simulink model "PubIfCommonEHRV2_MDL"  (R2020b)
settings: Solver=FixedStepAuto  StartTime=0.0  StopTime=Inf  RelTol=1e-3
PostLoadFcn:
  | if any(exist('dsrtsu_mdlpostloadfcn', 'file') ~= 0), dsrtsu_mdlpostloadfcn('Execute', bdroot); end
InitFcn:
  | , if any(exist('dsmpb_private', 'file') ~= 0), dsmpb_private('dsmpb_mdlclblib', 'Init', bdroot); end,
undefined symbols (not defined in the file): CAMERA_STATE_INITIAL, CAMERA_STATE_NORMAL, CURVATURE_UNKNOWN, DISTANCE_UNKONWN, DRIVING_ON_HIGHWAY_YES, EHR_CYCLE, FORWARD_LOOKING_DISTANCE_LIMIT, IFC_HUT_INTERFACE_NO_RESPONSE, IFC_HUT_INTERFACE_RESPONSE, MAP_DATA_VALID_VALID, MSG_TYPE_PROFILE_LONG, MSG_TYPE_PROFILE_SHORT, MSG_TYPE_SEGMENT, MSG_TYPE_STUB, OFFSET_INVALID, OFFSET_MAX, P_EHRV2_dCurvatureFar, P_EHRV2_dCurvatureMatrix, P_EHRV2_dSlopeFar, P_EHRV2_dSlopeMatrix, P_EHRV2_dVehForwardLooking, P_EHRV2_dVehRearLooking, P_EHRV2_tIFCHUTNoResponseOfForecastTreeReset, P_EHRV2_tIFCHUTNoResponseOfTimeout, P_EHRV2_tIFCHUTResponseTimeout, PROFILE_SHORT_NO_OTHER_VALUE, PROFILE_SHORT_TYPE_CURVATURE, PROFILE_SHORT_TYPE_SLOPE, REAR_LOOKING_DISTANCE_LIMIT, SLOPE_UNKNOWN, STUB_CMPLX_INSCT, STUB_FORM_OF_WAY_HIGH_RING_ROAD, STUB_FORM_OF_WAY_NORMAL_RING_ROAD
libraries: simulink x5
(part 2 of 4)

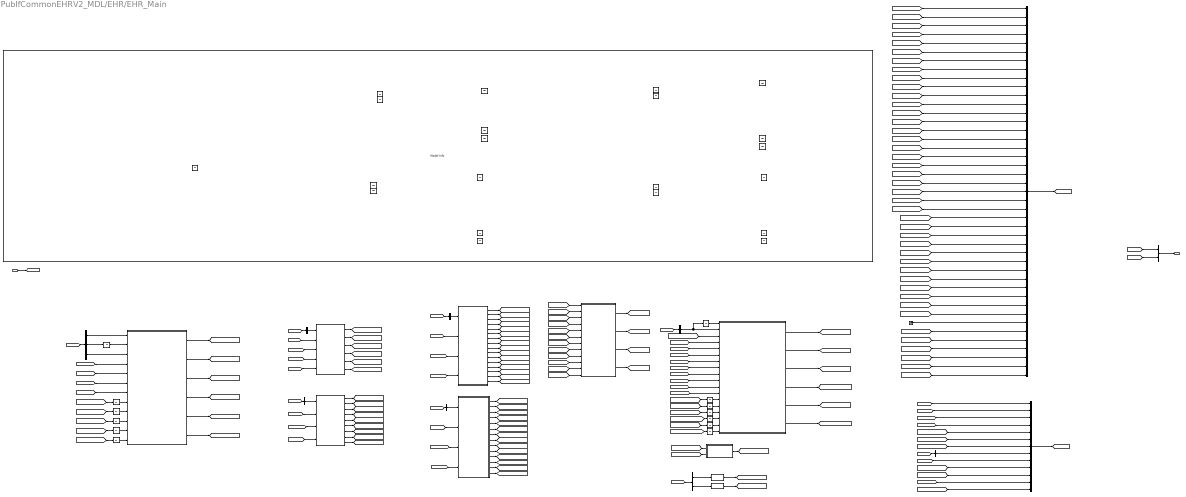
== system PubIfCommonEHRV2_MDL/EHR/EHR_Main ==
  EHR_InputData : Inport
  Bus Creator : BusCreator  Inputs=43
  Bus Creator1 : BusCreator  Inputs=13
  Bus Creator2 : BusCreator  Inputs=2
  Bus Selector : BusSelector  OutputSignals=PositionStruct,PositionStruct,StubStruct
  Bus Selector1 : BusSelector  OutputSignals=SegmentStruct
  Bus Selector10 : BusSelector  OutputSignals=PositionStruct,ProfileShortStruct
  Bus Selector11 : BusSelector  OutputSignals=PositionStruct,PositionStruct,ProfileShortStruct
  Bus Selector12 : BusSelector  OutputSignals=ProfileLongStruct
  Bus Selector13 : BusSelector  OutputSignals=PositionStruct,ProfileLongStruct
  Bus Selector14 : BusSelector  OutputSignals=PositionStruct,PositionStruct,ProfileLongStruct
  Bus Selector{6,8,15..16} (4 alike) : BusSelector  OutputSignals=PositionStruct
  Bus Selector17 : BusSelector  OutputSignals=OtherMessageStruct.ECU_State
  Bus Selector18 : BusSelector  OutputSignals=PositionStruct,PositionStruct,OtherMessageStruct.VehSpdDisp
  Bus Selector19 : BusSelector  OutputSignals=StubStruct
  Bus Selector2 : BusSelector  OutputSignals=StubStruct
  Bus Selector20 : BusSelector  OutputSignals=MetaDataStruct.MetaSpdUnits,MetaDataStruct.MetaCountryCode
  Bus Selector3 : BusSelector  OutputSignals=PositionStruct,StubStruct
  Bus Selector4 : BusSelector  OutputSignals=PositionStruct,SegmentStruct
  Bus Selector5 : BusSelector  OutputSignals=PositionStruct,PositionStruct,SegmentStruct
  Bus Selector7 : BusSelector  OutputSignals=SegmentStruct.SegMsgType
  Bus Selector9 : BusSelector  OutputSignals=ProfileShortStruct
  DR_Calc_IFCHUTInterface : MATLAB Function  TreatAsAtomicUnit=on
  DR_Calc_MapDataValid : MATLAB Function  TreatAsAtomicUnit=on
  DR_Calc_ProfileLongReconstruct : MATLAB Function  TreatAsAtomicUnit=on
  DR_Calc_ProfileShortReconstruct : MATLAB Function  TreatAsAtomicUnit=on
  DR_Calc_RampDistance : MATLAB Function  TreatAsAtomicUnit=on
  DR_Calc_SegmentReconstruct : MATLAB Function  TreatAsAtomicUnit=on
  DR_Calc_StubReconstruct : MATLAB Function  TreatAsAtomicUnit=on
  DS_Calc_ForecastTreeReset : MATLAB Function  TreatAsAtomicUnit=on
  DS_Calc_ProfileLongIsInDataWindow : MATLAB Function  TreatAsAtomicUnit=on
  DS_Calc_ProfileLongIsUpdated : MATLAB Function  TreatAsAtomicUnit=on
  DS_Calc_ProfileLongVector : MATLAB Function  TreatAsAtomicUnit=on
  DS_Calc_ProfileShortIsInDataWindow : MATLAB Function  TreatAsAtomicUnit=on
  DS_Calc_ProfileShortIsUpdated : MATLAB Function  TreatAsAtomicUnit=on
  DS_Calc_ProfileShortVector : MATLAB Function  TreatAsAtomicUnit=on
  DS_Calc_SegmentIsInDataWindow : MATLAB Function  TreatAsAtomicUnit=on
  DS_Calc_SegmentIsUpdated : MATLAB Function  TreatAsAtomicUnit=on
  DS_Calc_SegmentVector : MATLAB Function  TreatAsAtomicUnit=on
  DS_Calc_StubIsInDataWindow : MATLAB Function  TreatAsAtomicUnit=on
  DS_Calc_StubIsUpdated : MATLAB Function  TreatAsAtomicUnit=on
  DS_Calc_StubVector : MATLAB Function  TreatAsAtomicUnit=on
  Data Type Conversion : DataTypeConversion  OutDataTypeStr=uint8
  Data Type Conversion1 : DataTypeConversion  OutDataTypeStr=uint16
  Ground11 : Ground
  MATLAB Function : MATLAB Function  TreatAsAtomicUnit=on
  Model Info1 : simulink/Model-Wide Utilities/Model Info  Frame=on  DisplayStringWithTags=DS_Calc_SegmentVector  HorizontalTextAlignment=Left  LeftAlignmentValue=0.02
  Model Info2 : simulink/Model-Wide Utilities/Model Info  Frame=on  DisplayStringWithTags=DS_Calc_ProfileShortVector  HorizontalTextAlignment=Left  LeftAlignmentValue=0.02
  Model Info3 : simulink/Model-Wide Utilities/Model Info  Frame=on  DisplayStringWithTags=DS_Calc_StubVector  HorizontalTextAlignment=Left  LeftAlignmentValue=0.02
  Model Info4 : simulink/Model-Wide Utilities/Model Info  Frame=on  DisplayStringWithTags=DS_Calc_ProfileLongVector  HorizontalTextAlignment=Left  LeftAlignmentValue=0.02
  Model Info9 : simulink/Model-Wide Utilities/Model Info  Frame=on  DisplayStringWithTags=DS  HorizontalTextAlignment=Left  LeftAlignmentValue=0.02
  Unit Delay{,1..33} (34 alike) : UnitDelay  SampleTime=-1  HasFrameUpgradeWarning=on
  EHR_OutputData : Outport
  wires:
  DR_Calc_ProfileLongReconstruct/1(RampInDistance) -> [RampInDistance2]
  [IFCHUTInterfaceNoResponseFlag1] -> Unit Delay20/1
  Unit Delay6/1 -> DS_Calc_ProfileShortIsUpdated/2(ProfileShortVector)
  Bus Selector3/2 -> DS_Calc_StubIsInDataWindow/2(StubStruct)  "<StubStruct>"
  Unit Delay30/1 -> DS_Calc_ForecastTreeReset/2(StubStructK1)
  DS_Calc_StubVector/2(StubVectorSize) -> [StubVectorSize]  "EHRV2_StubVectorSize"
  [StubVectorSize] -> DR_Calc_StubReconstruct/3(StubVectorSize)
  Bus Selector18/2 -> Unit Delay31/1  "<PositionStruct>"
  Bus Selector19/1 -> Unit Delay30/1, DS_Calc_ForecastTreeReset/1(StubStruct)  "<StubStruct>"
  [PositionPathIdxInvalidCycles] -> Unit Delay29/1
  [SegmentVectorSize] -> Unit Delay15/1
  [MapDataValid] -> DR_Calc_ProfileLongReconstruct/4(MapDataValid)
  [MapDataValid] -> DR_Calc_ProfileShortReconstruct/4(MapDataValid)
  [SegmentVectorSize] -> DR_Calc_MapDataValid/5(SegmentVectorSize)
  DR_Calc_MapDataValid/3(PositionJumpOutOfRange) -> [PositionJumpOutOfRange]  "EHRV2_PositionJumpOutOfRange"
  Bus Selector3/1 -> DS_Calc_StubIsInDataWindow/1(PositionStruct)  "<PositionStruct>"
  [EHR_InputData] -> Bus Selector4/1
  [StubVectorSize] -> DS_Calc_ProfileShortVector/8(StubVectorSize)
  DS_Calc_ForecastTreeReset/1(ForecastTreeResetFlag) -> [ForecastTreeResetFlag]  "EHRV2_ForecastTreeResetFlag"
  Unit Delay8/1 -> DS_Calc_StubIsUpdated/3(StubVectorSize)
  [ProfileShortVectorSize] -> DR_Calc_MapDataValid/6(ProfileShortVectorSize)
  Bus Selector5/2 -> Unit Delay3/1  "<PositionStruct>"
  Bus Selector18/3 -> DR_Calc_MapDataValid/3(IPVehSpdDisp)  "<VehSpdDisp>"
  DR_Calc_MapDataValid/4(PositionJumpOutOfRangeCycles) -> [PositionJumpOutOfRangeCycles]  "EHRV2_PositionJumpOutOfRangeCycles"
  [ProfileLongIsUpdated] -> DS_Calc_ProfileLongVector/4(ProfileLongIsUpdated)
  [MapDataValid] -> DR_Calc_StubReconstruct/4(MapDataValid)
  [ForecastTreeResetFlag] -> Bus Creator1/12  "ForecastTreeResetFlag"
  DR_Calc_ProfileShortReconstruct/5(RoadSlopeFar) -> [RoadSlopeFar]
  [StubVectorSize] -> Unit Delay8/1
  [StubVectorSize] -> Unit Delay2/1
  Bus Selector13/1 -> DS_Calc_ProfileLongIsInDataWindow/1(PositionStruct)  "<PositionStruct>"
  [RoadSlopeMatrix] -> Bus Creator/35  "RoadSlopeMatrix"
  Unit Delay14/1 -> DS_Calc_SegmentIsUpdated/2(SegmentVector)
  [ForecastTreeResetFlag] -> DS_Calc_StubVector/6(ForecastTreeResetFlag)
  [StubVector] -> DR_Calc_StubReconstruct/2(StubVector)
  DR_Calc_ProfileShortReconstruct/6(RoadCurvatureMatrix) -> [RoadCurvatureMatrix]
  [NumOfLaneDrvDir] -> Bus Creator/10  "NumOfLaneDrvDir"
  DR_Calc_MapDataValid/2(PositionOffsetCycles) -> [PositionOffsetCycles]  "EHRV2_PositionOffsetCycles"
  [SegmentVector] -> DR_Calc_SegmentReconstruct/2(SegmentVector)
  [SegmentVectorSize] -> DR_Calc_SegmentReconstruct/3(SegmentVectorSize)
  Bus Selector1/1 -> DS_Calc_SegmentIsUpdated/1(SegmentStruct)  "<SegmentStruct>"
  Unit Delay13/1 -> DS_Calc_ProfileLongIsUpdated/2(ProfileLongVector)
  Unit Delay16/1 -> DS_Calc_ProfileLongIsUpdated/3(ProfileLongVectorSize)
  [ElectronicEyeSpeedLimit] -> Bus Creator/27  "ElectronicEyeSpeedLimit"
  [StubVector] -> DS_Calc_ProfileShortIsInDataWindow/3(StubVector)
  [SegmentIsInDataWindow] -> DS_Calc_SegmentVector/5(SegmentIsInDataWindow)
  [StubVector] -> DS_Calc_ProfileLongIsInDataWindow/3(StubVector)
  [StubVectorSize] -> DS_Calc_ProfileLongIsInDataWindow/4(StubVectorSize)
  [EHR_InputData] -> Bus Selector10/1
  [ProfileShortVector] -> Unit Delay6/1
  Bus Selector6/1 -> DR_Calc_SegmentReconstruct/1(PositionStruct)  "<PositionStruct>"
  Bus Selector5/3 -> DS_Calc_SegmentVector/3(SegmentStruct)  "<SegmentStruct>"
  DS_Calc_ProfileShortVector/2(ProfileShortVectorSize) -> [ProfileShortVectorSize]  "EHRV2_ProfileShortVectorSize"
  [PositionOffsetCycles] -> Unit Delay25/1
  Bus Selector9/1 -> DS_Calc_ProfileShortIsUpdated/1(ProfileShortStruct)  "<ProfileShortStruct>"
  DS_Calc_ProfileShortIsUpdated/1(ProfileShortIsUpdated) -> [ProfileShortIsUpdated]  "EHRV2_ProfileShortIsUpdated"
  DR_Calc_SegmentReconstruct/2(FormOfWay) -> [FormOfWay]
  DS_Calc_ProfileShortVector/1(ProfileShortVector) -> [ProfileShortVector]
  Unit Delay5/1 -> DS_Calc_SegmentVector/10(SegmentVectorSizeK1)
  [StubVectorSize] -> DR_Calc_MapDataValid/4(StubVectorSize)
  DR_Calc_SegmentReconstruct/6(SpeedLimit) -> [SpeedLimit]
  [StubVectorSize] -> DS_Calc_SegmentIsInDataWindow/4(StubVectorSize)
  Unit Delay4/1 -> DS_Calc_SegmentVector/9(SegmentVectorK1)
  [RoadSlopeFar] -> Bus Creator/32  "RoadSlopeFar"
  [StubVector] -> DS_Calc_ProfileShortVector/7(StubVector)
  [SpeedLimit] -> Bus Creator/23  "SpeedLimit"
  Bus Selector2/1 -> DS_Calc_StubIsUpdated/1(StubStruct)  "<StubStruct>"
  [StubVector] -> Unit Delay1/1
  DR_Calc_SegmentReconstruct/8(TunnelDistance) -> [TunnelDistance]
  Unit Delay3/1 -> DS_Calc_SegmentVector/2(PositionStructK1)
  [EHR_OutputSignals] -> Bus Creator2/1  "EHR_OutputSignals"
  Bus Selector5/1 -> DS_Calc_SegmentVector/1(PositionStruct)  "<PositionStruct>"
  Unit Delay/1 -> DS_Calc_StubVector/2(PositionStructK1)
  [EHR_InputData] -> Bus Selector5/1
  [SegmentVectorSize] -> Bus Creator1/2  "SegmentVectorSize"
  [RoadCurvatureFarDistance] -> Bus Creator/30  "RoadCurvatureFarDistance"
  EHR_InputData/1 -> [EHR_InputData]
  Unit Delay1/1 -> DS_Calc_StubVector/7(StubVectorK1)
  [EHR_DebugSignals] -> Bus Creator2/2  "EHR_DebugSignals"
  [IFCHUTInterface] -> Bus Creator/38  "IFCHUTInterface"
  DS_Calc_StubIsInDataWindow/1(StubIsInDataWindow) -> [StubIsInDataWindow]  "EHRV2_StubIsInDataWindow"
  [SegmentVectorSize] -> Unit Delay5/1
  [EHR_InputData] -> Bus Selector2/1
  DS_Calc_SegmentIsUpdated/1(SegmentIsUpdated) -> [SegmentIsUpdated]  "EHRV2_SegmentIsUpdated"
  [EHR_InputData] -> Bus Selector6/1
  [SegmentVector] -> Unit Delay4/1
  [EHR_InputData] -> Bus Selector3/1
  Unit Delay15/1 -> DS_Calc_SegmentIsUpdated/3(SegmentVectorSize)
  [EHR_InputData] -> Bus Selector/1
  [RoadCurvatureFar] -> Bus Creator/29  "RoadCurvatureFar"
  DS_Calc_SegmentVector/2(SegmentVectorSize) -> [SegmentVectorSize]  "EHRV2_SegmentVectorSize"
  [TunnelDistance] -> Bus Creator/3  "TunnelDistance"
  Bus Selector/2 -> Unit Delay/1  "<PositionStruct>"
  [FormOfWay] -> Bus Creator/2  "FormOfWay"
  Unit Delay2/1 -> DS_Calc_StubVector/8(StubVectorSizeK1)
  [StubVectorSize] -> DS_Calc_ProfileShortIsInDataWindow/4(StubVectorSize)
  [DrivingOnHighWay] -> Bus Creator/1  "DrivingOnHighWay"
  [ForecastTreeResetFlag] -> DS_Calc_ProfileShortVector/6(ForecastTreeResetFlag)
  Unit Delay29/1 -> DR_Calc_MapDataValid/12(PositionPathIdxInvalidCyclesK1)
  DR_Calc_SegmentReconstruct/4(EnterBridgeInfo) -> [EnterBridgeInfo]
  DS_Calc_ProfileLongIsUpdated/1(ProfileLongIsUpdated) -> [ProfileLongIsUpdated]  "EHRV2_ProfileLongIsUpdated"
  [EHR_InputData] -> Bus Selector11/1
  Bus Selector18/1 -> DR_Calc_MapDataValid/1(PositionStruct)  "<PositionStruct>"
  DS_Calc_StubVector/1(StubVector) -> [StubVector]
  DR_Calc_ProfileShortReconstruct/4(RoadSlope) -> [RoadSlope]
  [RoadCurvatureMatrixSize] -> Bus Creator/34  "RoadCurvatureMatrixSize"
  [StubVector] -> Unit Delay7/1
  DR_Calc_ProfileLongReconstruct/3(ElectronicEyeSpeedLimit) -> [ElectronicEyeSpeedLimit]
  [StubVector] -> DS_Calc_SegmentIsInDataWindow/3(StubVector)
  [EnterBridgeInfo] -> Bus Creator/6  "EnterBridgeInfo"
  DR_Calc_ProfileShortReconstruct/2(RoadCurvatureFar) -> [RoadCurvatureFar]
  DS_Calc_ProfileLongVector/2(ProfileLongVectorSize) -> [ProfileLongVectorSize]  "EHRV2_ProfileLongVectorSize"
  [PositionJumpOutOfRange] -> Unit Delay26/1
  [EHR_InputData] -> Bus Selector15/1
  [ProfileLongVectorSize] -> Unit Delay19/1
  Bus Selector4/1 -> DS_Calc_SegmentIsInDataWindow/1(PositionStruct)  "<PositionStruct>"
  Bus Selector10/1 -> DS_Calc_ProfileShortIsInDataWindow/1(PositionStruct)  "<PositionStruct>"
  Unit Delay10/1 -> DS_Calc_ProfileShortVector/2(PositionStructK1)
  Bus Selector16/1 -> DR_Calc_ProfileLongReconstruct/1(PositionStruct)  "<PositionStruct>"
  [SegmentIsUpdated] -> DS_Calc_SegmentVector/4(SegmentIsUpdated)
  [ProfileLongVectorSize] -> Unit Delay16/1
  Bus Selector15/1 -> DR_Calc_ProfileShortReconstruct/1(PositionStruct)  "<PositionStruct>"
  [EHR_InputData] -> Bus Selector14/1
  [ProfileShortVectorSize] -> DR_Calc_ProfileShortReconstruct/3(ProfileShortVectorSize)
  [StubVectorSize] -> DS_Calc_ProfileLongVector/8(StubVectorSize)
  [EHR_InputData] -> Bus Selector12/1
  [ProfileLongVector] -> Unit Delay13/1
  [ProfileLongVector] -> Unit Delay18/1
  [EHR_InputData] -> Bus Selector13/1
  [ProfileLongVector] -> DR_Calc_ProfileLongReconstruct/2(ProfileLongVector)
  DS_Calc_ProfileLongIsInDataWindow/1(ProfileLongIsInDataWindow) -> [ProfileLongIsInDataWindow]  "EHRV2_ProfileLongIsInDataWindow"
  Bus Selector8/1 -> DR_Calc_StubReconstruct/1(PositionStruct)  "<PositionStruct>"
  [SegmentIsUpdated] -> Bus Creator1/9  "SegmentIsUpdated"
  Unit Delay25/1 -> DR_Calc_MapDataValid/8(PositionOffsetCyclesK1)
  Bus Selector11/1 -> DS_Calc_ProfileShortVector/1(PositionStruct)  "<PositionStruct>"
  Unit Delay27/1 -> DR_Calc_MapDataValid/10(PositionJumpOutOfRangeCyclesK1)
  [RampDistance] -> Bus Creator/7  "RampDistance"
  Bus Selector10/2 -> DS_Calc_ProfileShortIsInDataWindow/2(ProfileShortStruct)  "<ProfileShortStruct>"
  DR_Calc_MapDataValid/1(MapDataValid) -> [MapDataValid]
  [ForecastTreeResetFlag] -> DS_Calc_ProfileLongVector/6(ForecastTreeResetFlag)
  [ProfileShortVectorSize] -> Unit Delay9/1
  DS_Calc_ProfileShortIsInDataWindow/1(ProfileShortIsInDataWindow) -> [ProfileShortIsInDataWindow]  "EHRV2_ProfileShortIsInDataWindow"
  [StubVector] -> DS_Calc_SegmentVector/7(StubVector)
  [RoadSlopeMatrixSize] -> Bus Creator/36  "RoadSlopeMatrixSize"
  [EHR_InputData] -> Bus Selector16/1
  [StubIsUpdated] -> DS_Calc_StubVector/4(StubIsUpdated)
  [ProfileShortVector] -> DR_Calc_ProfileShortReconstruct/2(ProfileShortVector)
  Bus Selector11/3 -> DS_Calc_ProfileShortVector/3(ProfileShortStruct)  "<ProfileShortStruct>"
  [PositionPathIdxInvalid] -> Unit Delay28/1
  Unit Delay9/1 -> DS_Calc_ProfileShortIsUpdated/3(ProfileShortVectorSize)
  [EHR_InputData] -> Bus Selector17/1
  DS_Calc_SegmentVector/1(SegmentVector) -> [SegmentVector]
  DS_Calc_SegmentIsInDataWindow/1(SegmentIsInDataWindow) -> [SegmentIsInDataWindow]  "EHRV2_SegmentIsInDataWindow"
  Bus Selector14/3 -> DS_Calc_ProfileLongVector/3(ProfileLongStruct)  "<ProfileLongStruct>"
  DR_Calc_MapDataValid/6(PositionPathIdxInvalidCycles) -> [PositionPathIdxInvalidCycles]  "EHRV2_PositionPathIdxInvalidCycles"
  Unit Delay17/1 -> DS_Calc_ProfileLongVector/2(PositionStructK1)
  DR_Calc_ProfileShortReconstruct/7(RoadCurvatureMatrixSize) -> [RoadCurvatureMatrixSize]
  Unit Delay19/1 -> DS_Calc_ProfileLongVector/10(ProfileLongVectorSizeK1)
  DR_Calc_ProfileShortReconstruct/8(RoadSlopeMatrix) -> [RoadSlopeMatrix]
  [IFCHUTInterfaceNoResponseFlag2] -> Bus Creator1/7  "IFCHUTInterfaceNoResponseFlag2"
  Bus Selector13/2 -> DS_Calc_ProfileLongIsInDataWindow/2(ProfileLongStruct)  "<ProfileLongStruct>"
  [EHR_InputData] -> Bus Selector1/1
  DR_Calc_IFCHUTInterface/6(IFCHUTInterfaceNoResponseFlag2Cycles) -> [IFCHUTInterfaceNoResponseFlag2Cycles]  "EHRV2_IFCHUTInterfaceNoResponseFlag2Cycles"
  [SegmentVectorSize] -> DR_Calc_IFCHUTInterface/6(SegmentVectorSize)
  [StubVectorSize] -> DS_Calc_SegmentVector/8(StubVectorSize)
  [EHR_InputData] -> Bus Selector9/1
  DR_Calc_SegmentReconstruct/3(EnterTunnelInfo) -> [EnterTunnelInfo]
  Unit Delay18/1 -> DS_Calc_ProfileLongVector/9(ProfileLongVectorK1)
  Bus Selector14/2 -> Unit Delay17/1  "<PositionStruct>"
  DR_Calc_SegmentReconstruct/9(BridgeDistance) -> [BridgeDistance]
  [ProfileShortVector] -> Unit Delay11/1
  [StubVectorSize] -> DR_Calc_IFCHUTInterface/4(StubVectorSize)
  [IFCHUTInterfaceNoResponseFlag2Cycles] -> Unit Delay24/1
  DS_Calc_ProfileLongVector/1(ProfileLongVector) -> [ProfileLongVector]
  DR_Calc_IFCHUTInterface/5(IFCHUTInterfaceNoResponseFlag2) -> [IFCHUTInterfaceNoResponseFlag2]  "EHRV2_IFCHUTInterfaceNoResponseFlag2"
  Bus Selector17/1 -> Unit Delay33/1, DR_Calc_IFCHUTInterface/2(ECU_State)  "<ECU_State>"
  [EHR_InputData] -> Bus Selector7/1
  [SegmentVector] -> Unit Delay14/1
  Unit Delay12/1 -> DS_Calc_ProfileShortVector/10(ProfileShortVectorSizeK1)
  [EnterTunnelInfo] -> Bus Creator/4  "EnterTunnelInfo"
  DR_Calc_IFCHUTInterface/3(IFCHUTInterfaceNoResponseFlag1) -> [IFCHUTInterfaceNoResponseFlag1]  "EHRV2_IFCHUTInterfaceNoResponseFlag1"
  Bus Selector7/1 -> Bus Creator1/8  "<SegMsgType>"
  DR_Calc_ProfileShortReconstruct/1(RoadCurvature) -> [RoadCurvature]
  [ProfileShortVectorSize] -> Unit Delay12/1
  Bus Creator1/1 -> [EHR_DebugSignals]
  Bus Selector11/2 -> Unit Delay10/1  "<PositionStruct>"
  [ProfileLongVectorSize] -> DR_Calc_IFCHUTInterface/10(ProfileLongVectorSize)
  DR_Calc_ProfileShortReconstruct/3(RoadCurvatureFarDistance) -> [RoadCurvatureFarDistance]
  DS_Calc_StubIsUpdated/1(StubIsUpdated) -> [StubIsUpdated]  "EHRV2_StubIsUpdated"
  [ProfileShortVectorSize] -> DR_Calc_IFCHUTInterface/8(ProfileShortVectorSize)
  Unit Delay26/1 -> DR_Calc_MapDataValid/9(PositionJumpOutOfRangeK1)
  [IFCHUTInterfaceNoResponseFlag1] -> Bus Creator1/6  "IFCHUTInterfaceNoResponseFlag1"
  [RoadSlope] -> Bus Creator/31  "RoadSlope"
  [ProfileLongIsInDataWindow] -> DS_Calc_ProfileLongVector/5(ProfileLongIsInDataWindow)
  [StubVector] -> DS_Calc_ProfileLongVector/7(StubVector)
  [BridgeDistance] -> Bus Creator/5  "BridgeDistance"
  [IFCHUTInterfaceNoResponseFlag2] -> Unit Delay23/1
  DR_Calc_StubReconstruct/1(RampOutDistance) -> [RampOutDistance]
  DR_Calc_SegmentReconstruct/1(DrivingOnHighWay) -> [DrivingOnHighWay]
  Unit Delay28/1 -> DR_Calc_MapDataValid/11(PositionPathIdxInvalidK1)
  [ProfileLongVectorSize] -> DR_Calc_ProfileLongReconstruct/3(ProfileLongVectorSize)
  DR_Calc_ProfileLongReconstruct/2(ElectronicEyeDistance) -> [ElectronicEyeDistance]
  [EHR_InputData] -> Bus Selector8/1
  Bus Selector/1 -> DS_Calc_StubVector/1(PositionStruct)  "<PositionStruct>"
  DR_Calc_MapDataValid/5(PositionPathIdxInvalid) -> [PositionPathIdxInvalid]  "EHRV2_PositionPathIdxInvalid"
  [ProfileLongVectorSize] -> DR_Calc_MapDataValid/7(ProfileLongVectorSize)
  [IFCHUTInterface] -> Unit Delay21/1
  Bus Selector/3 -> DS_Calc_StubVector/3(StubStruct)  "<StubStruct>"
  DR_Calc_IFCHUTInterface/2(IFCHUTInterfaceCycles) -> [IFCHUTInterfaceCycles]  "EHRV2_IFCHUTInterfaceCycles"
  [IFCHUTInterfaceCycles] -> Unit Delay22/1
  [StubVectorSize] -> Bus Creator1/1  "StubVectorSize"
  [ProfileShortVectorSize] -> Bus Creator1/3  "ProfileShortVectorSize"
  [ProfileShortIsInDataWindow] -> DS_Calc_ProfileShortVector/5(ProfileShortIsInDataWindow)
  [ForecastTreeResetFlag] -> DS_Calc_SegmentVector/6(ForecastTreeResetFlag)
  Unit Delay31/1 -> DR_Calc_MapDataValid/2(PositionStructK1)
  [ElectronicEyeDistance] -> Bus Creator/26  "ElectronicEyeDistance"
  [RampOutDistance] -> DR_Calc_RampDistance/2(RampOutDistance)
  [PositionJumpOutOfRangeCycles] -> Bus Creator1/11  "PositionJumpOutOfRangeCycles"
  [RoadCurvature] -> Bus Creator/28  "RoadCurvature"
  DR_Calc_IFCHUTInterface/1(IFCHUTInterface) -> [IFCHUTInterface]
  [IFCHUTInterfaceNoResponseFlag1Cycles] -> Unit Delay32/1
  [RampInDistance] -> DR_Calc_RampDistance/1(RampInDistance)
  [EHR_InputData] -> Bus Selector18/1
  [PositionOffsetCycles] -> Bus Creator1/10  "PositionOffsetCycles"
  Bus Creator2/1 -> EHR_OutputData/1
  DR_Calc_IFCHUTInterface/4(IFCHUTInterfaceNoResponseFlag1Cycles) -> [IFCHUTInterfaceNoResponseFlag1Cycles]  "EHRV2_IFCHUTInterfaceNoResponseFlag1Cycles"
  [IFCHUTInterfaceCycles] -> Bus Creator1/5  "IFCHUTInterfaceCycles"
  [ProfileShortIsUpdated] -> DS_Calc_ProfileShortVector/4(ProfileShortIsUpdated)
  Bus Selector4/2 -> DS_Calc_SegmentIsInDataWindow/2(SegmentStruct)  "<SegmentStruct>"
  DR_Calc_ProfileShortReconstruct/9(RoadSlopeMatrixSize) -> [RoadSlopeMatrixSize]
  Unit Delay7/1 -> DS_Calc_StubIsUpdated/2(StubVector)
  [RoadCurvatureMatrix] -> Bus Creator/33  "RoadCurvatureMatrix"
  DR_Calc_RampDistance/1(RampDistance) -> [RampDistance]
  [PositionJumpOutOfRangeCycles] -> Unit Delay27/1
  DR_Calc_SegmentReconstruct/5(NumOfLaneDrvDir) -> [NumOfLaneDrvDir]
  Bus Selector14/1 -> DS_Calc_ProfileLongVector/1(PositionStruct)  "<PositionStruct>"
  Bus Selector12/1 -> DS_Calc_ProfileLongIsUpdated/1(ProfileLongStruct)  "<ProfileLongStruct>"
  [EHR_InputData] -> Bus Selector19/1
  [MapDataValid] -> Bus Creator/39  "MapDataValid"
  [StubIsInDataWindow] -> DS_Calc_StubVector/5(StubIsInDataWindow)
  [ProfileLongVectorSize] -> Bus Creator1/4  "ProfileLongVectorSize"
  Unit Delay11/1 -> DS_Calc_ProfileShortVector/9(ProfileShortVectorK1)
  [MapDataValid] -> DR_Calc_SegmentReconstruct/4(MapDataValid)
  [ForecastTreeResetFlag] -> DR_Calc_IFCHUTInterface/12(ForecastTreeResetFlag)
  Unit Delay21/1 -> DR_Calc_IFCHUTInterface/13(IFCHUTInterfaceK1)
  Unit Delay22/1 -> DR_Calc_IFCHUTInterface/14(IFCHUTInterfaceCyclesK1)
  Unit Delay20/1 -> DR_Calc_IFCHUTInterface/15(IFCHUTInterfaceNoResponseFlag1K1)
  Unit Delay32/1 -> DR_Calc_IFCHUTInterface/16(IFCHUTInterfaceNoResponseFlag1CyclesK1)
  Unit Delay23/1 -> DR_Calc_IFCHUTInterface/17(IFCHUTInterfaceNoResponseFlag2K1)
  Unit Delay24/1 -> DR_Calc_IFCHUTInterface/18(IFCHUTInterfaceNoResponseFlag2CyclesK1)
  [StubVector] -> DR_Calc_IFCHUTInterface/5(StubVector)
  [SegmentVector] -> DR_Calc_IFCHUTInterface/7(SegmentVector)
  [ProfileShortVector] -> DR_Calc_IFCHUTInterface/9(ProfileShortVector)
  [ProfileLongVector] -> DR_Calc_IFCHUTInterface/11(ProfileLongVector)
  [DrivingOnHighWay] -> DR_Calc_IFCHUTInterface/3(DrivingOnHighWay)
  [RampInDistance] -> Bus Creator/8  "RampInDistance"
  [RampOutDistance] -> Bus Creator/9  "RampOutDistance"
  DR_Calc_ProfileLongReconstruct/4(TrafficSignDistance) -> [TrafficSignDistance]
  DR_Calc_ProfileLongReconstruct/5(TrafficSignValue) -> [TrafficSignValue]
  [TrafficSignDistance] -> Bus Creator/11  "TrafficSignDistance"
  [TrafficSignValue] -> Bus Creator/12  "TrafficSignValue"
  DR_Calc_StubReconstruct/2(RingRoadOutDistance) -> [RingRoadOutDistance]
  [RingRoadOutDistance] -> Bus Creator1/13  "RingRoadOutDistance"
  Unit Delay33/1 -> DR_Calc_IFCHUTInterface/1(ECU_StateK1)
  [EHR_InputData] -> Bus Selector20/1
  Bus Selector20/1 -> Data Type Conversion/1  "<MetaSpdUnits>"
  Data Type Conversion/1 -> [SpeedUnit]
  [SpeedUnit] -> Bus Creator/25  "SpeedUnit"
  DR_Calc_ProfileLongReconstruct/6(WeatherTypeValue) -> [WeatherTypeValue]
  [WeatherTypeValue] -> Bus Creator/13  "WeatherTypeValue"
  [Temperature] -> Bus Creator/14  "Temperature"
  [TrafficJamDistanceHold] -> Bus Creator/16  "TrafficJamDistanceHold"
  [TrafficJamDistance] -> Bus Creator/15  "TrafficJamDistance"
  [FuncRoadClass] -> Bus Creator/19  "FuncRoadClass"
  [BuildUpArea] -> Bus Creator/20  "BuildUpArea"
  [CtrlPointDistance] -> Bus Creator/18  "CtrlPointDistance"
  [RepairRoadPointDistance] -> Bus Creator/17  "RepairRoadPointDistance"
  [CmplxInsctDistance] -> Bus Creator/21  "CmplxInsctDistance"
  [SpeedLimitType] -> Bus Creator/24  "SpeedLimitType"
  [CountryCode] -> Bus Creator/22  "CountryCode"
  Bus Creator/1 -> [EHR_OutputSignals]
  Ground11/1 -> Bus Creator/37  "MultiWayIntersectionDistance"
  Bus Selector20/2 -> Data Type Conversion1/1  "<MetaCountryCode>"
  Data Type Conversion1/1 -> [CountryCode]
  DR_Calc_StubReconstruct/3(CmplxInsctDistance) -> [CmplxInsctDistance]
  DR_Calc_SegmentReconstruct/7(SpeedLimitType) -> [SpeedLimitType]
  DR_Calc_SegmentReconstruct/10(FuncRoadClass) -> [FuncRoadClass]
  DR_Calc_SegmentReconstruct/11(BuildUpArea) -> [BuildUpArea]
  DR_Calc_ProfileLongReconstruct/7(Temperature) -> [Temperature]
  DR_Calc_ProfileLongReconstruct/8(TrafficJamDistance) -> [TrafficJamDistance]
  DR_Calc_ProfileLongReconstruct/9(TrafficJamDistanceHold) -> [TrafficJamDistanceHold]
  DR_Calc_ProfileLongReconstruct/10(RepairRoadPointDistance) -> [RepairRoadPointDistance]
  DR_Calc_ProfileLongReconstruct/11(CtrlPointDistance) -> [CtrlPointDistance]
  DR_Calc_StubReconstruct/4(StubRamp_dirc1) -> [StubRamp_dirc1]
  [StubRamp_dirc] -> Bus Creator/40  "StubRamp_dirc"
  [SegmentVector] -> DR_Calc_StubReconstruct/5(SegmentVector)
  DR_Calc_StubReconstruct/5(Stub_Type1) -> [Stub_Type1]
  DR_Calc_StubReconstruct/6(Ramp_Type1) -> [Ramp_Type1]
  DR_Calc_SegmentReconstruct/13(Stub_Type3) -> [Stub_Type3]
  DR_Calc_SegmentReconstruct/14(Ramp_Type3) -> [Ramp_Type3]
  DR_Calc_SegmentReconstruct/12(StubRamp_dirc3) -> [StubRamp_dirc3]
  DR_Calc_SegmentReconstruct/15(RampInDistance) -> [RampInDistance1]
  DR_Calc_ProfileLongReconstruct/12(StubRamp_dirc2) -> [StubRamp_dirc2]
  DR_Calc_ProfileLongReconstruct/13(Stub_Type2) -> [Stub_Type2]
  DR_Calc_ProfileLongReconstruct/14(Ramp_Type2) -> [Ramp_Type2]
  [RampInDistance1] -> MATLAB Function/2(RampInDistance1)
  [RampInDistance2] -> MATLAB Function/3(RampInDistance2)
  [Stub_Type1] -> MATLAB Function/4(Stub_Type1)
  [Stub_Type2] -> MATLAB Function/5(Stub_Type2)
  [Stub_Type3] -> MATLAB Function/6(Stub_Type3)
  [Ramp_Type1] -> MATLAB Function/7(Ramp_Type1)
  [Ramp_Type2] -> MATLAB Function/8(Ramp_Type2)
  [Ramp_Type3] -> MATLAB Function/9(Ramp_Type3)
  [StubRamp_dirc1] -> MATLAB Function/10(StubRamp_dirc1)
  [StubRamp_dirc2] -> MATLAB Function/11(StubRamp_dirc2)
  [StubRamp_dirc3] -> MATLAB Function/12(StubRamp_dirc3)
  MATLAB Function/1(StubRamp_dirc) -> [StubRamp_dirc]
  MATLAB Function/2(RampInDistance) -> [RampInDistance]
  MATLAB Function/3(Stub_Type) -> [Stub_Type]
  MATLAB Function/4(Ramp_Type) -> [Ramp_Type]
  [RampOutDistance] -> MATLAB Function/1(RampOutDistance)
  DR_Calc_SegmentReconstruct/16(OnNavPath) -> [OnNavPath]
  [Stub_Type] -> Bus Creator/41  "Stub_Type"
  [Ramp_Type] -> Bus Creator/42  "Ramp_Type"
  [OnNavPath] -> Bus Creator/43  "OnNavPath"

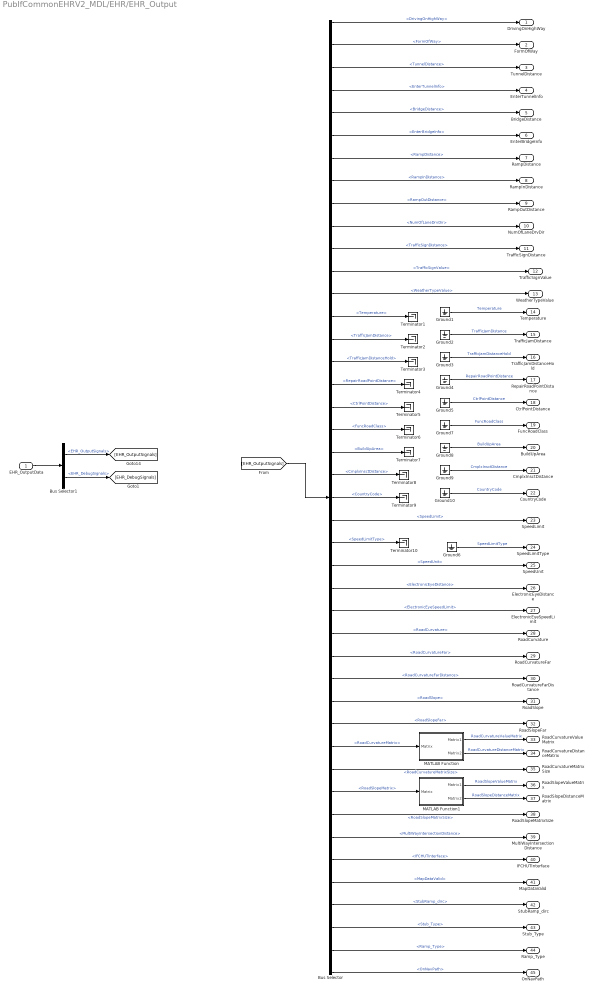
== system PubIfCommonEHRV2_MDL/EHR/EHR_Output ==
  EHR_OutputData : Inport
  Bus Selector : BusSelector  OutputSignals=DrivingOnHighWay,FormOfWay,TunnelDistance,EnterTunnelInfo,BridgeDistance,EnterBridgeInfo,RampDistance,RampInDistance,RampOutDistance,NumOfLaneDrvDir,TrafficSignDistance,TrafficSignValue,WeatherTypeValue,Temperature,TrafficJamDistance,TrafficJamDistanceHold,RepairRoadPointDistance,CtrlPointDistance,FuncRoadClass,BuildUpArea,CmplxInsctDistance,CountryCode,SpeedLimit,SpeedLimitType,SpeedUnit,ElectronicEyeDistance,ElectronicEyeSpeedLimit,RoadCurvature,RoadCurvatureFar,RoadCurvatureFarDistance,RoadSlope,RoadSlopeFar,RoadCurvatureMatrix,RoadCurvatureMatrixSize,RoadSlopeMatrix,RoadSlopeMatrixSize,MultiWayIntersectionDistance,IFCHUTInterface,MapDataValid,StubRamp_dirc,Stub_Type,Ramp_Type,OnNavPath
  Bus Selector1 : BusSelector  OutputSignals=EHR_OutputSignals,EHR_DebugSignals
  Ground{1..10} (10 alike) : Ground
  MATLAB Function : MATLAB Function  TreatAsAtomicUnit=on
  MATLAB Function1 : MATLAB Function  TreatAsAtomicUnit=on
  Terminator{1..10} (10 alike) : Terminator
  DrivingOnHighWay : Outport
  FormOfWay : Outport  Port=2
  TunnelDistance : Outport  Port=3
  EnterTunnelInfo : Outport  Port=4
  BridgeDistance : Outport  Port=5
  EnterBridgeInfo : Outport  Port=6
  RampDistance : Outport  Port=7
  RampInDistance : Outport  Port=8
  RampOutDistance : Outport  Port=9
  NumOfLaneDrvDir : Outport  Port=10
  TrafficSignDistance : Outport  Port=11
  TrafficSignValue : Outport  Port=12
  WeatherTypeValue : Outport  Port=13
  Temperature : Outport  Port=14
  TrafficJamDistance : Outport  Port=15
  TrafficJamDistanceHold : Outport  Port=16
  RepairRoadPointDistance : Outport  Port=17
  CtrlPointDistance : Outport  Port=18
  FuncRoadClass : Outport  Port=19
  BuildUpArea : Outport  Port=20
  CmplxInsctDistance : Outport  Port=21
  CountryCode : Outport  Port=22
  SpeedLimit : Outport  Port=23
  SpeedLimitType : Outport  Port=24
  SpeedUnit : Outport  Port=25
  ElectronicEyeDistance : Outport  Port=26
  ElectronicEyeSpeedLimit : Outport  Port=27
  RoadCurvature : Outport  Port=28
  RoadCurvatureFar : Outport  Port=29
  RoadCurvatureFarDistance : Outport  Port=30
  RoadSlope : Outport  Port=31
  RoadSlopeFar : Outport  Port=32
  RoadCurvatureValueMatrix : Outport  Port=33
  RoadCurvatureDistanceMatrix : Outport  Port=34
  RoadCurvatureMatrixSize : Outport  Port=35
  RoadSlopeValueMatrix : Outport  Port=36
  RoadSlopeDistanceMatrix : Outport  Port=37
  RoadSlopeMatrixSize : Outport  Port=38
  MultiWayIntersectionDistance : Outport  Port=39
  IFCHUTInterface : Outport  Port=40
  MapDataValid : Outport  Port=41
  StubRamp_dirc : Outport  Port=42
  Stub_Type : Outport  Port=43
  Ramp_Type : Outport  Port=44
  OnNavPath : Outport  Port=45
  wires:
  EHR_OutputData/1 -> Bus Selector1/1
  Bus Selector1/1 -> [EHR_OutputSignals]  "<EHR_OutputSignals>"
  Bus Selector1/2 -> [EHR_DebugSignals]  "<EHR_DebugSignals>"
  [EHR_OutputSignals] -> Bus Selector/1
  Bus Selector/33 -> MATLAB Function/1(Matrix)  "<RoadCurvatureMatrix>"
  Bus Selector/35 -> MATLAB Function1/1(Matrix)  "<RoadSlopeMatrix>"
  Bus Selector/1 -> DrivingOnHighWay/1  "<DrivingOnHighWay>"
  Bus Selector/2 -> FormOfWay/1  "<FormOfWay>"
  Bus Selector/3 -> TunnelDistance/1  "<TunnelDistance>"
  Bus Selector/4 -> EnterTunnelInfo/1  "<EnterTunnelInfo>"
  Bus Selector/5 -> BridgeDistance/1  "<BridgeDistance>"
  Bus Selector/6 -> EnterBridgeInfo/1  "<EnterBridgeInfo>"
  Bus Selector/7 -> RampDistance/1  "<RampDistance>"
  Bus Selector/8 -> RampInDistance/1  "<RampInDistance>"
  Bus Selector/9 -> RampOutDistance/1  "<RampOutDistance>"
  Bus Selector/10 -> NumOfLaneDrvDir/1  "<NumOfLaneDrvDir>"
  Bus Selector/11 -> TrafficSignDistance/1  "<TrafficSignDistance>"
  Bus Selector/12 -> TrafficSignValue/1  "<TrafficSignValue>"
  Bus Selector/24 -> Terminator10/1  "<SpeedLimitType>"
  Bus Selector/25 -> SpeedUnit/1  "<SpeedUnit>"
  Bus Selector/26 -> ElectronicEyeDistance/1  "<ElectronicEyeDistance>"
  Bus Selector/27 -> ElectronicEyeSpeedLimit/1  "<ElectronicEyeSpeedLimit>"
  Bus Selector/28 -> RoadCurvature/1  "<RoadCurvature>"
  Bus Selector/29 -> RoadCurvatureFar/1  "<RoadCurvatureFar>"
  Bus Selector/30 -> RoadCurvatureFarDistance/1  "<RoadCurvatureFarDistance>"
  Bus Selector/31 -> RoadSlope/1  "<RoadSlope>"
  Bus Selector/32 -> RoadSlopeFar/1  "<RoadSlopeFar>"
  MATLAB Function/1(Matrix1) -> RoadCurvatureValueMatrix/1  "RoadCurvatureValueMatrix"
  MATLAB Function/2(Matrix2) -> RoadCurvatureDistanceMatrix/1  "RoadCurvatureDistanceMatrix"
  Bus Selector/34 -> RoadCurvatureMatrixSize/1  "<RoadCurvatureMatrixSize>"
  MATLAB Function1/1(Matrix1) -> RoadSlopeValueMatrix/1  "RoadSlopeValueMatrix"
  MATLAB Function1/2(Matrix2) -> RoadSlopeDistanceMatrix/1  "RoadSlopeDistanceMatrix"
  Bus Selector/36 -> RoadSlopeMatrixSize/1  "<RoadSlopeMatrixSize>"
  Bus Selector/38 -> IFCHUTInterface/1  "<IFCHUTInterface>"
  Bus Selector/39 -> MapDataValid/1  "<MapDataValid>"
  Ground1/1 -> Temperature/1  "Temperature"
  Ground3/1 -> TrafficJamDistanceHold/1  "TrafficJamDistanceHold"
  Ground2/1 -> TrafficJamDistance/1  "TrafficJamDistance"
  Ground7/1 -> FuncRoadClass/1  "FuncRoadClass"
  Ground5/1 -> CtrlPointDistance/1  "CtrlPointDistance"
  Ground4/1 -> RepairRoadPointDistance/1  "RepairRoadPointDistance"
  Ground8/1 -> BuildUpArea/1  "BuildUpArea"
  Ground10/1 -> CountryCode/1  "CountryCode"
  Ground9/1 -> CmplxInsctDistance/1  "CmplxInsctDistance"
  Bus Selector/13 -> WeatherTypeValue/1  "<WeatherTypeValue>"
  Bus Selector/14 -> Terminator1/1  "<Temperature>"
  Bus Selector/16 -> Terminator3/1  "<TrafficJamDistanceHold>"
  Bus Selector/15 -> Terminator2/1  "<TrafficJamDistance>"
  Bus Selector/20 -> Terminator7/1  "<BuildUpArea>"
  Bus Selector/19 -> Terminator6/1  "<FuncRoadClass>"
  Bus Selector/18 -> Terminator5/1  "<CtrlPointDistance>"
  Bus Selector/17 -> Terminator4/1  "<RepairRoadPointDistance>"
  Bus Selector/23 -> SpeedLimit/1  "<SpeedLimit>"
  Bus Selector/22 -> Terminator9/1  "<CountryCode>"
  Bus Selector/21 -> Terminator8/1  "<CmplxInsctDistance>"
  Ground6/1 -> SpeedLimitType/1  "SpeedLimitType"
  Bus Selector/37 -> MultiWayIntersectionDistance/1  "<MultiWayIntersectionDistance>"
  Bus Selector/40 -> StubRamp_dirc/1  "<StubRamp_dirc>"
  Bus Selector/41 -> Stub_Type/1  "<Stub_Type>"
  Bus Selector/42 -> Ramp_Type/1  "<Ramp_Type>"
  Bus Selector/43 -> OnNavPath/1  "<OnNavPath>"

== matlab function PubIfCommonEHRV2_MDL/EHR/EHR_Main/MATLAB Function ==
  data: RampOutDistance input; StubRamp_dirc output; RampInDistance1 input; RampInDistance2 input; Stub_Type1 input; Stub_Type2 input; Stub_Type3 input; Ramp_Type1 input; Ramp_Type2 input; Ramp_Type3 input; StubRamp_dirc1 input; StubRamp_dirc2 input; StubRamp_dirc3 input; RampInDistance output; Stub_Type output; Ramp_Type output; DISTANCE_UNKONWN parameter
function [StubRamp_dirc,RampInDistance,Stub_Type,Ramp_Type] = fcn(RampOutDistance,RampInDistance1,RampInDistance2,Stub_Type1,Stub_Type2,Stub_Type3,Ramp_Type1,Ramp_Type2,Ramp_Type3,StubRamp_dirc1,StubRamp_dirc2,StubRamp_dirc3, DISTANCE_UNKONWN)
    StubRamp_dirc = uint8(0);
    RampInDistance = DISTANCE_UNKONWN;
    Stub_Type = uint8(0);
    Ramp_Type = uint8(0);
    %不存在汇出工况
if RampOutDistance == DISTANCE_UNKONWN
    %匝道汇入与右侧有车辆汇入工况
    if RampInDistance1 < RampInDistance2
        StubRamp_dirc = StubRamp_dirc3;
        RampInDistance = RampInDistance1;
        Stub_Type = Stub_Type3;
        Ramp_Type = Ramp_Type3;
    end
    if RampInDistance1 > RampInDistance2
        StubRamp_dirc = StubRamp_dirc2;
        RampInDistance = RampInDistance2;
        Stub_Type = Stub_Type2;
        Ramp_Type = Ramp_Type2;
    end
    if (RampInDistance1 == RampInDistance2) && (RampInDistance1 < DISTANCE_UNKONWN)
        StubRamp_dirc = StubRamp_dirc3;
        RampInDistance = RampInDistance1;
        Stub_Type = Stub_Type3;
        Ramp_Type = Ramp_Type3;
    end
    if (RampInDistance1 == RampInDistance2) && (RampInDistance1 == DISTANCE_UNKONWN)
        StubRamp_dirc = uint8(0);
        RampInDistance = DISTANCE_UNKONWN;
        Stub_Type = uint8(0);
        Ramp_Type = uint8(0);
    end
else
    %存在汇出口工况
    if (RampInDistance1 == DISTANCE_UNKONWN) && (RampInDistance2 == DISTANCE_UNKONWN) 
        StubRamp_dirc = StubRamp_dirc1;
        RampInDistance = DISTANCE_UNKONWN;
        Stub_Type = Stub_Type1;
        Ramp_Type = Ramp_Type1;
    end
    if (RampInDistance1 < DISTANCE_UNKONWN) && (RampInDistance1 < RampInDistance2) && (RampOutDistance < RampInDistance1) 
        StubRamp_dirc = StubRamp_dirc1;
        RampInDistance = RampInDistance1;
        Stub_Type = Stub_Type1;
        Ramp_Type = Ramp_Type1;
    end
    if (RampInDistance1 < DISTANCE_UNKONWN) && (RampInDistance1 < RampInDistance2) && (RampOutDistance > RampInDistance1) 
        StubRamp_dirc = StubRamp_dirc3;
        RampInDistance = RampInDistance1;
        Stub_Type = Stub_Type3;
        Ramp_Type = Ramp_Type3;
    end
    if (RampInDistance2 < DISTANCE_UNKONWN) && (RampInDistance2 < RampInDistance1) && (RampOutDistance < RampInDistance2) 
        StubRamp_dirc = StubRamp_dirc1;
        RampInDistance = RampInDistance2;
        Stub_Type = Stub_Type1;
        Ramp_Type = Ramp_Type1;
    end
    if (RampInDistance2 < DISTANCE_UNKONWN) && (RampInDistance2 < RampInDistance1) && (RampOutDistance > RampInDistance2) 
        StubRamp_dirc = StubRamp_dirc2;
        RampInDistance = RampInDistance2;
        Stub_Type = Stub_Type2;
        Ramp_Type = Ramp_Type2;
    end
end

== matlab function PubIfCommonEHRV2_MDL/EHR/EHR_Input/EHR_Calc_ProfileLongPreCheck ==
  data: PositionStructIn input Bus: PositionStruct; ProfileLongStructIn input Bus: ProfileLongStruct; ProfileLongStructOut output Bus: ProfileLongStruct; ProfileLongStructOutK1 input Bus: ProfileLongStruct; MSG_TYPE_PROFILE_LONG parameter; OFFSET_INVALID parameter; REAR_LOOKING_DISTANCE_LIMIT parameter; FORWARD_LOOKING_DISTANCE_LIMIT parameter; OFFSET_MAX parameter
function ProfileLongStructOut = fcn(PositionStructIn,ProfileLongStructIn,ProfileLongStructOutK1, ...
    MSG_TYPE_PROFILE_LONG, OFFSET_INVALID, REAR_LOOKING_DISTANCE_LIMIT, FORWARD_LOOKING_DISTANCE_LIMIT, OFFSET_MAX)

if ProfileLongStructIn.ProfLongMsgType == MSG_TYPE_PROFILE_LONG
    ProfileLongStructOut = ProfileLongStructIn;
    ProfileLongStructOut.ProfLongRelativeOffset = EHR_Calc_RelativeOffset(PositionStructIn,...
        ProfileLongStructIn.ProfLongPathIdx,ProfileLongStructIn.ProfLongOffset);
else
    ProfileLongStructOut = ProfileLongStructOutK1;
end

== matlab function PubIfCommonEHRV2_MDL/EHR/EHR_Input/EHR_Calc_ProfileShortPreCheck ==
  data: PositionStructIn input Bus: PositionStruct; ProfileShortStructIn input Bus: ProfileShortStruct; ProfileShortStructOut output Bus: ProfileShortStruct; ProfileShortStructOutK1 input Bus: ProfileShortStruct; MSG_TYPE_PROFILE_SHORT parameter; OFFSET_INVALID parameter; REAR_LOOKING_DISTANCE_LIMIT parameter; FORWARD_LOOKING_DISTANCE_LIMIT parameter; OFFSET_MAX parameter
function ProfileShortStructOut = fcn(PositionStructIn,ProfileShortStructIn,ProfileShortStructOutK1, ...
    MSG_TYPE_PROFILE_SHORT, OFFSET_INVALID, REAR_LOOKING_DISTANCE_LIMIT, FORWARD_LOOKING_DISTANCE_LIMIT, OFFSET_MAX)

if ProfileShortStructIn.ProfShortMsgType == MSG_TYPE_PROFILE_SHORT
    ProfileShortStructOut = ProfileShortStructIn;
    ProfileShortStructOut.ProfShortRelativeOffset = EHR_Calc_RelativeOffset(PositionStructIn,...
        ProfileShortStructIn.ProfShortPathIdx,ProfileShortStructIn.ProfShortOffset);
else
    ProfileShortStructOut = ProfileShortStructOutK1;
end

== matlab function PubIfCommonEHRV2_MDL/EHR/EHR_Input/EHR_Calc_SegmentPreCheck ==
  data: PositionStructIn input Bus: PositionStruct; SegmentStructIn input Bus: SegmentStruct; SegmentStructOut output Bus: SegmentStruct; SegmentStructOutK1 input Bus: SegmentStruct; MSG_TYPE_SEGMENT parameter; OFFSET_INVALID parameter; REAR_LOOKING_DISTANCE_LIMIT parameter; FORWARD_LOOKING_DISTANCE_LIMIT parameter; OFFSET_MAX parameter
function SegmentStructOut = fcn(PositionStructIn,SegmentStructIn,SegmentStructOutK1, ...
    MSG_TYPE_SEGMENT, OFFSET_INVALID, REAR_LOOKING_DISTANCE_LIMIT, FORWARD_LOOKING_DISTANCE_LIMIT, OFFSET_MAX)

if SegmentStructIn.SegMsgType == MSG_TYPE_SEGMENT
    SegmentStructOut = SegmentStructIn;
    SegmentStructOut.SegRelativeOffset = EHR_Calc_RelativeOffset(PositionStructIn,...
        SegmentStructIn.SegPathIdx,SegmentStructIn.SegOffset);
else
    SegmentStructOut = SegmentStructOutK1;
end

== matlab function PubIfCommonEHRV2_MDL/EHR/EHR_Input/EHR_Calc_StubPreCheck ==
  data: PositionStructIn input Bus: PositionStruct; StubStructIn input Bus: StubStruct; StubStructOut output Bus: StubStruct; StubStructOutK1 input Bus: StubStruct; MSG_TYPE_STUB parameter; OFFSET_INVALID parameter; REAR_LOOKING_DISTANCE_LIMIT parameter; FORWARD_LOOKING_DISTANCE_LIMIT parameter; OFFSET_MAX parameter
function StubStructOut = fcn(PositionStructIn,StubStructIn,StubStructOutK1, ...
    MSG_TYPE_STUB, OFFSET_INVALID, REAR_LOOKING_DISTANCE_LIMIT, FORWARD_LOOKING_DISTANCE_LIMIT, OFFSET_MAX)

if StubStructIn.StubMsgType == MSG_TYPE_STUB
    StubStructOut = StubStructIn;
    StubStructOut.StubRelativeOffset = EHR_Calc_RelativeOffset(PositionStructIn,...
        StubStructIn.StubPathIdx,StubStructIn.StubOffset);
else
    StubStructOut = StubStructOutK1;
end

== matlab function PubIfCommonEHRV2_MDL/EHR/EHR_Input/EHR_Calc_VehSpdDisp ==
  data: VehSpd input; VehSpdDisp output single
function VehSpdDisp = fcn(VehSpd)

VehSpdDisp = single(VehSpd * 1.03 + 1.3);

== matlab function PubIfCommonEHRV2_MDL/EHR/EHR_Main/DR_Calc_IFCHUTInterface ==
  data: ECU_StateK1 input; ECU_State input; DrivingOnHighWay input; StubVectorSize input; StubVector input; SegmentVectorSize input; SegmentVector input; ProfileShortVectorSize input; ProfileShortVector input; ProfileLongVectorSize input; ProfileLongVector input; ForecastTreeResetFlag input; IFCHUTInterfaceK1 input; IFCHUTInterfaceCyclesK1 input; IFCHUTInterfaceNoResponseFlag1K1 input; IFCHUTInterfaceNoResponseFlag1CyclesK1 input; IFCHUTInterfaceNoResponseFlag2K1 input; IFCHUTInterfaceNoResponseFlag2CyclesK1 input; P_EHRV2_tIFCHUTResponseTimeout parameter; P_EHRV2_tIFCHUTNoResponseOfTimeout parameter; P_EHRV2_tIFCHUTNoResponseOfForecastTreeReset parameter; EHR_CYCLE parameter; IFC_HUT_INTERFACE_RESPONSE parameter; IFC_HUT_INTERFACE_NO_RESPONSE parameter; CAMERA_STATE_INITIAL parameter; IFCHUTInterface output uint8; IFCHUTInterfaceCycles output uint16; IFCHUTInterfaceNoResponseFlag1 output boolean; IFCHUTInterfaceNoResponseFlag1Cycles output uint16; IFCHUTInterfaceNoResponseFlag2 output boolean; IFCHUTInterfaceNoResponseFlag2Cycles output uint16; DRIVING_ON_HIGHWAY_YES parameter; CAMERA_STATE_NORMAL parameter
function [IFCHUTInterface, IFCHUTInterfaceCycles, IFCHUTInterfaceNoResponseFlag1, IFCHUTInterfaceNoResponseFlag1Cycles, IFCHUTInterfaceNoResponseFlag2, IFCHUTInterfaceNoResponseFlag2Cycles]...
    = fcn(ECU_StateK1,ECU_State,DrivingOnHighWay,...
    StubVectorSize, StubVector, SegmentVectorSize, SegmentVector, ProfileShortVectorSize, ProfileShortVector, ProfileLongVectorSize, ProfileLongVector, ForecastTreeResetFlag,...
    IFCHUTInterfaceK1, IFCHUTInterfaceCyclesK1,...
    IFCHUTInterfaceNoResponseFlag1K1, IFCHUTInterfaceNoResponseFlag1CyclesK1,...
    IFCHUTInterfaceNoResponseFlag2K1, IFCHUTInterfaceNoResponseFlag2CyclesK1,...
    P_EHRV2_tIFCHUTResponseTimeout, P_EHRV2_tIFCHUTNoResponseOfTimeout, P_EHRV2_tIFCHUTNoResponseOfForecastTreeReset, EHR_CYCLE, IFC_HUT_INTERFACE_RESPONSE, IFC_HUT_INTERFACE_NO_RESPONSE, CAMERA_STATE_INITIAL,  DRIVING_ON_HIGHWAY_YES, CAMERA_STATE_NORMAL)

IFCHUTInterfaceNoResponseFlag1 = IFCHUTInterfaceNoResponseFlag1K1;
IFCHUTInterfaceNoResponseFlag2 = IFCHUTInterfaceNoResponseFlag2K1;

%%%%IFC HUT Interface%%%%
if (0 == StubVectorSize)...
&& (0 == SegmentVectorSize)...
&& (0 == ProfileShortVectorSize)...
&& (0 == ProfileLongVectorSize)
    IFCHUTInterface = IFC_HUT_INTERFACE_RESPONSE;
elseif SegmentVectorSize >= length(SegmentVector)   %Segment Oversize(New Requirement)
    IFCHUTInterface = IFC_HUT_INTERFACE_RESPONSE;
elseif ((StubVectorSize >= length(StubVector)) || (ProfileShortVectorSize >= length(ProfileShortVector)) || (ProfileLongVectorSize >= length(ProfileLongVector)))...   %Other Vector Oversize and DriveOnHighway(New Requirement)
    && (DrivingOnHighWay == DRIVING_ON_HIGHWAY_YES)
    IFCHUTInterface = IFC_HUT_INTERFACE_RESPONSE;
else
    IFCHUTInterface = IFC_HUT_INTERFACE_NO_RESPONSE;
end

%IFCHUTInterface should be suppressed while camera state initial to normal
if CAMERA_STATE_INITIAL == ECU_State
    IFCHUTInterface = IFC_HUT_INTERFACE_NO_RESPONSE;
elseif (CAMERA_STATE_INITIAL == ECU_StateK1) && (CAMERA_STATE_NORMAL == ECU_State)
    IFCHUTInterface = IFC_HUT_INTERFACE_RESPONSE;
end

%IFCHUTInterface should be suppressed 5 cycles in this case
IFCHUTInterfaceCycles = EHR_Calc_Duration_Cycles(IFCHUTInterface,IFCHUTInterfaceK1,IFCHUTInterfaceCyclesK1);
if (IFC_HUT_INTERFACE_RESPONSE == IFCHUTInterface)...
    && (IFCHUTInterfaceCycles >= (P_EHRV2_tIFCHUTResponseTimeout/EHR_CYCLE))
    IFCHUTInterfaceNoResponseFlag1 = true;
    IFCHUTInterfaceNoResponseFlag1CyclesK1 = uint16(0);   %IFCHUTInterfaceNoResponseFlag1CyclesK1 should be calculated from 0 again while IFCHUTInterfaceNoResponseFlag1 = true
end
IFCHUTInterfaceNoResponseFlag1Cycles = EHR_Calc_Duration_Cycles(IFCHUTInterfaceNoResponseFlag1,IFCHUTInterfaceNoResponseFlag1K1,IFCHUTInterfaceNoResponseFlag1CyclesK1);
if true == IFCHUTInterfaceNoResponseFlag1
    IFCHUTInterface = IFC_HUT_INTERFACE_NO_RESPONSE;
    if IFCHUTInterfaceNoResponseFlag1Cycles >= (P_EHRV2_tIFCHUTNoResponseOfTimeout/EHR_CYCLE)
        IFCHUTInterfaceNoResponseFlag1 = false;   %suppressed 5 cycles timeout
    end
end

%IFCHUTInterface should be suppressed 1s in this case
if true == ForecastTreeResetFlag
    IFCHUTInterfaceNoResponseFlag2 = true;
    IFCHUTInterfaceNoResponseFlag2CyclesK1 = uint16(0);
end
IFCHUTInterfaceNoResponseFlag2Cycles = EHR_Calc_Duration_Cycles(IFCHUTInterfaceNoResponseFlag2,IFCHUTInterfaceNoResponseFlag2K1,IFCHUTInterfaceNoResponseFlag2CyclesK1);
if true == IFCHUTInterfaceNoResponseFlag2
    IFCHUTInterface = IFC_HUT_INTERFACE_NO_RESPONSE;
    if IFCHUTInterfaceNoResponseFlag2Cycles >= (P_EHRV2_tIFCHUTNoResponseOfForecastTreeReset/EHR_CYCLE)
        IFCHUTInterfaceNoResponseFlag2 = false;   %suppressed 1s timeout
    end
end

== matlab function PubIfCommonEHRV2_MDL/EHR/EHR_Main/DR_Calc_MapDataValid ==
  data: PositionStruct input; PositionStructK1 input; IPVehSpdDisp input; StubVectorSize input; SegmentVectorSize input; ProfileShortVectorSize input; ProfileLongVectorSize input; PositionOffsetCyclesK1 input; PositionJumpOutOfRangeK1 input; PositionJumpOutOfRangeCyclesK1 input; PositionPathIdxInvalidK1 input; PositionPathIdxInvalidCyclesK1 input; P_EHRV2_dPositionJumpOutOfRangeForMapDataValid parameter; P_EHRV2_tPositionOffsetInvalidForMapDataValid parameter; P_EHRV2_tPositionJumpOutOfRangeForMapDataValid parameter; P_EHRV2_tPositionOffsetNotUpdateForMapDataValid parameter; P_EHRV2_vVehSpeedHighForMapDataValid parameter; P_EHRV2_tPositionPathIdxInvalidForMapDataValid parameter; MAP_DATA_VALID_INVALID parameter; MAP_DATA_VALID_VALID parameter; OFFSET_INVALID parameter; MapDataValid output uint8; PositionOffsetCycles output uint16; PositionJumpOutOfRange output boolean; PositionJumpOutOfRangeCycles output uint16; PositionPathIdxInvalid output boolean; PositionPathIdxInvalidCycles output uint16; EHR_CYCLE parameter
function [MapDataValid, PositionOffsetCycles, PositionJumpOutOfRange, PositionJumpOutOfRangeCycles, PositionPathIdxInvalid, PositionPathIdxInvalidCycles]...
    = fcn(PositionStruct, PositionStructK1,...
    IPVehSpdDisp,...
    StubVectorSize, SegmentVectorSize, ProfileShortVectorSize, ProfileLongVectorSize,...
    PositionOffsetCyclesK1, PositionJumpOutOfRangeK1, PositionJumpOutOfRangeCyclesK1, PositionPathIdxInvalidK1, PositionPathIdxInvalidCyclesK1,...
    P_EHRV2_dPositionJumpOutOfRangeForMapDataValid, P_EHRV2_tPositionOffsetInvalidForMapDataValid, P_EHRV2_tPositionJumpOutOfRangeForMapDataValid, P_EHRV2_tPositionOffsetNotUpdateForMapDataValid, P_EHRV2_vVehSpeedHighForMapDataValid, P_EHRV2_tPositionPathIdxInvalidForMapDataValid, MAP_DATA_VALID_INVALID, MAP_DATA_VALID_VALID, OFFSET_INVALID, EHR_CYCLE)

%%%%Map Data Valid%%%%
PositionOffsetCycles = EHR_Calc_Duration_Cycles(PositionStruct.PosnOffset,PositionStructK1.PosnOffset,PositionOffsetCyclesK1);

if abs(PositionStruct.PosnOffset - PositionStructK1.PosnOffset) > P_EHRV2_dPositionJumpOutOfRangeForMapDataValid
    PositionJumpOutOfRange = true;
else
    PositionJumpOutOfRange = false;
end
PositionJumpOutOfRangeCycles = EHR_Calc_Duration_Cycles(PositionJumpOutOfRange,PositionJumpOutOfRangeK1,PositionJumpOutOfRangeCyclesK1);

if (PositionStruct.PosnPathIdx >= 0) && (PositionStruct.PosnPathIdx <= 3)
    PositionPathIdxInvalid = true;
else
    PositionPathIdxInvalid = false;
end
PositionPathIdxInvalidCycles = EHR_Calc_Duration_Cycles(PositionPathIdxInvalid,PositionPathIdxInvalidK1,PositionPathIdxInvalidCyclesK1);

%Vector is null
if (0 == StubVectorSize)...
&& (0 == SegmentVectorSize)...
&& (0 == ProfileShortVectorSize)...
&& (0 == ProfileLongVectorSize)
    MapDataValid = MAP_DATA_VALID_INVALID;
    
%Position Offset Invalid Timeout
elseif (OFFSET_INVALID == PositionStruct.PosnOffset)...
    && (PositionOffsetCycles >= (P_EHRV2_tPositionOffsetInvalidForMapDataValid/EHR_CYCLE))
    MapDataValid = MAP_DATA_VALID_INVALID;

%%%EHR Do Not Monitor The Failure,The Functions Will Monitor The Failure By
%%%Themselives
% %Position/Meta CycCnt Failure
% elseif (true == Position_CycCnt_Failure) || (true == Meta_CycCnt_Failure)
%     MapDataValid = MAP_DATA_VALID_INVALID;
% 
% %Position/Meta ECU Timeout Failure
% elseif (true == Position_Timeout_Failure) || (true == Meta_Timeout_Failure)
%     MapDataValid = MAP_DATA_VALID_INVALID;

%Position Offset Jump Timeout
elseif (true == PositionJumpOutOfRange)...
    && (PositionJumpOutOfRangeCycles >= (P_EHRV2_tPositionJumpOutOfRangeForMapDataValid/EHR_CYCLE))
    MapDataValid = MAP_DATA_VALID_INVALID;
    
%Position Offset Not Update While Vehicle Speed High
elseif (IPVehSpdDisp > P_EHRV2_vVehSpeedHighForMapDataValid)...
    && (PositionOffsetCycles >= (P_EHRV2_tPositionOffsetNotUpdateForMapDataValid/EHR_CYCLE))
    MapDataValid = MAP_DATA_VALID_INVALID;
    
%Position Path ID Invalid Timeout
elseif (true == PositionPathIdxInvalid)...
    && (PositionPathIdxInvalidCycles >= (P_EHRV2_tPositionPathIdxInvalidForMapDataValid/EHR_CYCLE))
    MapDataValid = MAP_DATA_VALID_INVALID;
    
else
    MapDataValid = MAP_DATA_VALID_VALID;
end
